simulink library "vmc"  (R2021b)
settings: Solver=VariableStepAuto  StartTime=0.0  StopTime=10.0  RelTol=1e-3
undefined symbols (not defined in the file): AVMC_ACCDeltaTqGradeGn_X_deg, AVMC_ACCDeltaTqIGain4OVRD_X_kph, AVMC_ACCDeltaTqIGain4OVRD_Y_mps2, AVMC_ACCDeltaTqIGain_X_kph, AVMC_ACCDeltaTqIGain_Y_mps2, AVMC_ACCDeltaTqPGain_X_kph, AVMC_ACCDeltaTqPGain_Y_kph, AVMC_ACCGradeofst_X_G, AVMC_ACCGradeofst_Y_pct, AVMC_ACCLoSpdTqLoLim4JP_X_kph, AVMC_ACCLoSpdTqLoLim4JP_Y_deg, AVMC_ACCLoSpdTqLowerLim_X_kph, AVMC_ACCLoSpdTqLowerLim_Y_deg, AVMC_ACCReqAccelGain_X_mps2, AVMC_ACCReqAccelGain_Y_enum, AVMC_ADSPosGFBDeltaTq_X_kph, AVMC_ADSPosGFBDeltaTq_Y_mps2, AVMC_AggressJerkPCT4AT_X_kph, AVMC_AggressJerkPCT_X_kph, AVMC_AggressLimitPCT4AT_X_kph, AVMC_AggressLimitPCT_X_kph, AVMC_DECGradeofst_X_G, AVMC_DECGradeofst_Y_pct, AVMC_DISCDeltaTqIGain_X_kph, AVMC_DISCDeltaTqIGain_Y_mps2, AVMC_DISCDeltaTqPGain_X_kph, AVMC_DISCDeltaTqPGain_Y_kph, AVMC_EPSForceSelect_X_enum, AVMC_EPSForceSelect_Y_enum, AVMC_EPSForceSelectD21_X_enum, AVMC_EPSForceSelectD21_Y_enum, AVMC_ESCRegenOut_X_kph, AVMC_ESCRegenOut_Y_Deg, AVMC_ESCRegenOutEnSpd_X_Deg, AVMC_EstPitchSlopeTs_X_kph, AVMC_GradeCompFlt_X_kph, AVMC_GyroYBandLo_X_Gps, AVMC_HoldResTq_X_kph, AVMC_ISOAccLimit_X_mps, AVMC_ISODecLimit_X_mps, AVMC_ISOJerk_X_mps, AVMC_LatESCRegenOut_X_kph, AVMC_LatESCRegenOut_Y_Deg, AVMC_LongAccDeadZone_X_kph, AVMC_LongAccFiltTsforP2_X_Gps, AVMC_MCPresBaseTq_X_bar, AVMC_MSAPedalOvrd_X_kph, AVMC_MSASpdBand_X_kph, AVMC_MSATqDownEndTq_X_kph, AVMC_MSATqDownTime_X_kph, AVMC_NegZCHoldTq_X_kph, AVMC_OPDDisSlideRate_X_Deg, AVMC_OVRD2ActSR2FCMCMD_X_mps2, AVMC_PedalTqRWhlRatio_X_Nm, AVMC_PedalTqRWhlRatio_Y_gps, AVMC_PedalTqRWhlSlipGain_X_rat, AVMC_PedalTqRWhlSlipGain_Y_kph, AVMC_PedalTqRWhSTRGGain_X_deg, AVMC_PedalTqRWhSTRGGain_Y_kph, AVMC_PosZCHoldTq_X_kph ... (+593)
libraries: hcu_lib x143, simulink x96, tqr x4, $bdroot x1, simulink_extras x1
(part 4 of 17)

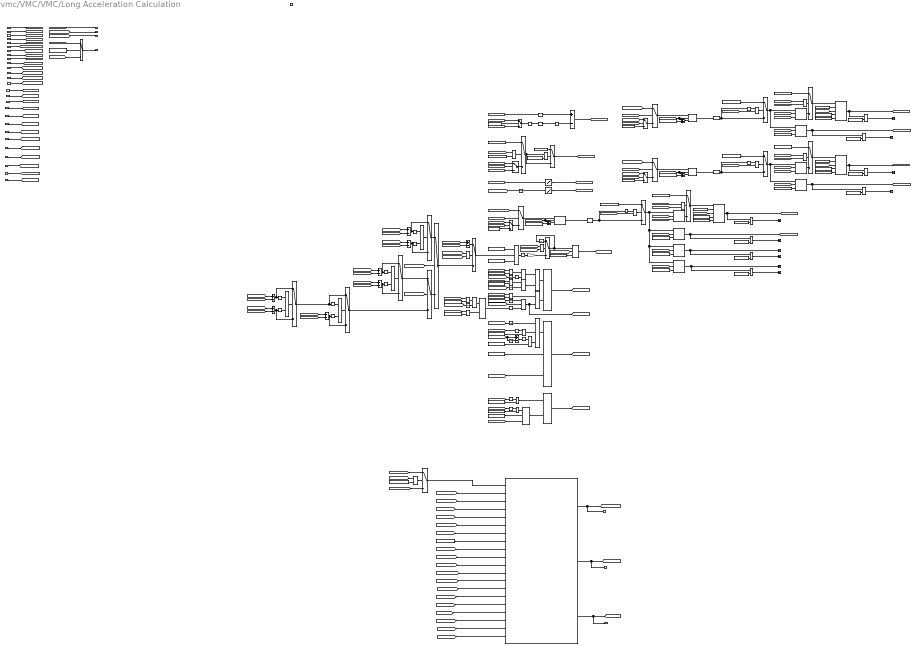
== system vmc/VMC/VMC/Long Acceleration Calculation ==
  VINP_GRADE_Deg : Inport
  VINP_LongAccel_Gps : Inport  Port=2
  VVMC_VehicleSpeed_kph : Inport  Port=3
  task_time_s : Inport  Port=4
  VVMC_EstSlopeCal_Deg : Inport  Port=5
  VVMC_LongAccelCalcuByVehSpdRaw_gps : Inport  Port=6
  VINP_DIDGetDynoMode_flg : Inport  Port=7
  VDDM_ESC5Err_flg : Inport  Port=8
  VINP_LongAccelV_flg : Inport  Port=9
  VINP_ACCRequiredAccel_mps2 : Inport  Port=10
  VVMC_LongAccelCalcuFrWhlRaw_gps : Inport  Port=11
  VVMC_LongAccelCalcuRrWhlRaw_gps : Inport  Port=12
  VVMC_FrWhlSpdInvalid_flg : Inport  Port=13
  VVMC_RrWhlSpdInvalid_flg : Inport  Port=14
  VVMC_CalibratedGyroY_Dps : Inport  Port=15
  VVMC_CalibratedAccX_G : Inport  Port=16
  VVMC_CalibratedAccY_G : Inport  Port=17
  VVMC_CalibratedAccZ_G : Inport  Port=18
  VINP_BrkPedalPos_pct : Inport  Port=19
  VTQD_GearActualPosn_enum : Inport  Port=20
  VDHP_ActAPSPosn_pct : Inport  Port=21
  VTQD_RegenMode_enum : Inport  Port=22
  VTQD_VehActSpd_kph : Inport  Port=23
  VTQD_PreLoadPreEn_flg : Inport  Port=24
  VTQR_RrTMTqReq_Nm : Inport  Port=25
  VTQR_FrTMTqReq_Nm : Inport  Port=26
  VPMM_DrivetrainSelect_enum : Inport  Port=27
  function : TriggerPort  TriggerType=function-call  VariantControl=(inherit)
  AND : Logic  Inputs=3  AllPortsSameDT=off  OutDataTypeStr=boolean
  AND1 : Logic  Operator=OR  AllPortsSameDT=off  OutDataTypeStr=boolean
  AND{2,5..8} (5 alike) : Logic  AllPortsSameDT=off  OutDataTypeStr=boolean
  AND3 : Logic  Operator=OR  AllPortsSameDT=off  OutDataTypeStr=boolean
  AND4 : Logic  Inputs=3  AllPortsSameDT=off  OutDataTypeStr=boolean
  Abs{,1..14} (15 alike) : Abs
  Add{,1..2,5..8,10..12} (10 alike) : Sum  Inputs=+-
  Add3 : Sum
  Add4 : Sum
  Add9 : Sum
  Asin1 : Trigonometry  Operator=asin
  Cast To Single{,1..4} (5 alike) : DataTypeConversion  OutDataTypeStr=single
  Constant : Constant  Value=KVMC_GradeSourceSW_flg
  Constant{1,8,17,22,24..25,33,36..37,40..41,44,47..48} (14 alike) : Constant  Value=ZERO_FLOAT
  Constant10 : Constant  Value=KVMC_LongAccelIncSRLim_gps2
  Constant11 : Constant  Value=KVMC_LongAccelDecSRLim_gps2
  Constant12 : Constant  Value=KVMC_EstSlopeFreezeSpd_kph
  Constant13 : Constant  Value=KVMC_EstSlopeUnFreezeSpd_kph
  Constant14 : Constant  Value=KVMC_EstSlopeTs_c
  Constant15 : Constant  Value=KVMC_EstSlope0SpdFreezeTime_s
  Constant16 : Constant  Value=KVMC_EstSlopeFreezeSpd_kph
  Constant18 : Constant  Value=KVMC_LongAccel0Boundary_Gps
  Constant19 : Constant  Value=KVMC_DIDGetDynoModeSW_flg
  Constant2 : Constant  Value=KVMC_AccBWFilCOFreqLo_raw32
  Constant20 : Constant  Value=KVMC_IMUGxStableThrs_Gps
  Constant21 : Constant  Value=KVMC_LongAccelSWSpd_kph
  Constant23 : Constant  Value=KVMC_GradeInvalidValue_deg
  Constant26 : Constant  Value=KVMC_EstSlopeUnFreezeSpd_kph
  Constant27 : Constant  Value=KVMC_AccBWFilterCutOffFreq_raw32
  Constant28 : Constant  Value=MINUSONE_FLOAT
  Constant29 : Constant  Value=ONE_FLOAT
  Constant3 : Constant  Value=KVMC_AccBWFilCOFreqMed_raw32
  Constant30 : Constant  Value=KVMC_EstSlopeFreezeAccel_Gps
  Constant31 : Constant  Value=KVMC_EstSlopeUnFreezeAccel_Gps
  Constant32 : Constant  Value=KVMC_EstSlopeAclUnFreezeTime_s
  Constant34 : Constant  Value=KVMC_LongAccelIncSRLim_gps2
  Constant35 : Constant  Value=KVMC_LongAccelDecSRLim_gps2
  Constant38 : Constant  Value=KVMC_AccBWFilterCutOffFreq_raw32
  Constant{5..7,9,39,46,50,52} (8 alike) : Constant  Value=KVMC_GravityValue_mps2
  Constant4 : Constant  Value=KVMC_AccBWFilCOFreqHigh_raw32
  Constant42 : Constant  Value=KVMC_LongAccelIncSRLim_gps2
  Constant43 : Constant  Value=KVMC_LongAccelDecSRLim_gps2
  Constant45 : Constant  Value=KVMC_AccBWFilterCutOffFreq_raw32
  Constant49 : Constant  Value=KVMC_AccBWFilCOFreqLo_raw32
  Constant51 : Constant  Value=KVMC_AccBWFilCOFreqLo_raw32
  Constant53 : Constant  Value=KVMC_EstSlopeGxSource_flg
  Constant54 : Constant  Value=C_TASK_10MS_S
  Constant55 : Constant  Value=KVMC_GradeTest_flg
  Degrees to Radians1 : simulink_extras/Transformations/Degrees to Radians
  DelayEnable : hcu_lib/Basic_Blocks/DelayEnable
  DelayEnable1 : hcu_lib/Basic_Blocks/DelayEnable
  Estimate Slope1 : Subsystem
  FirstOrderFilter{,1..11} (12 alike) : hcu_lib/Basic_Blocks/FirstOrderFilter
  Gain1 : Gain  Gain=RAD2DEG
  Logical Operator : Logic  Operator=OR  AllPortsSameDT=off  OutDataTypeStr=boolean
  Logical Operator1 : Logic  Operator=OR  AllPortsSameDT=off  OutDataTypeStr=boolean
  Logical Operator2 : Logic  Operator=OR  AllPortsSameDT=off  OutDataTypeStr=boolean
  MVMC_LongAccDeadZone_Y_Gps : Lookup_n-D  NumberOfTableDimensions=1  BreakpointsForDimension1=AVMC_LongAccDeadZone_X_kph  Table=MVMC_LongAccDeadZone_Y_Gps  InternalRulePriority=Speed  RndMeth=Simplest  InputSameDT=on
  MVMC_LongAccFiltTsforP2_Y_c : Lookup_n-D  NumberOfTableDimensions=1  BreakpointsForDimension1=AVMC_LongAccFiltTsforP2_X_Gps  Table=MVMC_LongAccFiltTsforP2_Y_c  InternalRulePriority=Speed  RndMeth=Simplest  InputSameDT=on
  NOT1 : Logic  Operator=NOT  AllPortsSameDT=off  OutDataTypeStr=boolean
  NOT2 : Logic  Operator=NOT  AllPortsSameDT=off  OutDataTypeStr=boolean
  OR : Logic  Operator=OR  AllPortsSameDT=off  OutDataTypeStr=boolean
  OR21 : Logic  AllPortsSameDT=off  OutDataTypeStr=boolean
  Product{1..7,15} (8 alike) : Product
  RateLimit1 : tqr/TQR/Determine Torque Request/TorqueArbitrament/TorqueSmooth/RateLimit
  RateLimit2 : tqr/TQR/Determine Torque Request/TorqueArbitrament/TorqueSmooth/RateLimit
  RateLimit3 : tqr/TQR/Determine Torque Request/TorqueArbitrament/TorqueSmooth/RateLimit
  Relational Operator : RelationalOperator  Operator=>  OutDataTypeStr=boolean  RndMeth=Simplest
  Relational Operator{1,4,7,10} (4 alike) : RelationalOperator  Operator=<  OutDataTypeStr=boolean  RndMeth=Simplest
  Relational Operator{2,5..6,11..12,124..127} (9 alike) : RelationalOperator  Operator=<=  OutDataTypeStr=boolean  RndMeth=Simplest
  Relational Operator3 : RelationalOperator  OutDataTypeStr=boolean  RndMeth=Simplest
  Relational Operator8 : RelationalOperator  OutDataTypeStr=boolean  RndMeth=Simplest
  Relational Operator9 : RelationalOperator  OutDataTypeStr=boolean  RndMeth=Simplest
  SR_Latch : hcu_lib/Basic_Blocks/SR_Latch
  SR_Latch1 : hcu_lib/Basic_Blocks/SR_Latch
  SR_Latch2 : hcu_lib/Basic_Blocks/SR_Latch
  Saturation Dynamic3 : simulink/Discontinuities/Saturation Dynamic  OutMin=[]  OutMax=[]  OutDataTypeStr=Inherit: Same as second input  OutDataType=fixdt(1, 16)  OutScaling=2^-10  DoSatur=off
  Sin1 : Trigonometry
  Switch{,1..4,6..8,10,12..14,16..17,82..83,85..89} (21 alike) : Switch  Criteria=u2 > Threshold
  Switch{5,9,11,15} (4 alike) : Switch  Criteria=u2 > Threshold  Threshold=KVMC_LongAccelSWSpd_kph
  Switch18 : Switch  Criteria=u2 ~= 0
      settings: AttributesFormatString=%<Criteria>
  Terminator{1..7,9..11} (10 alike) : Terminator
  Unit Delay{,1..7} (8 alike) : UnitDelay  SampleTime=-1  HasFrameUpgradeWarning=on
  VVMC_LongAcc_Gps : Outport
  VVMC_EstSlope_Deg : Outport  Port=2
  VVMC_LongAccFrWhl_Gps : Outport  Port=3
  VVMC_LongAccRrWhl_Gps : Outport  Port=4
  VVMC_EstSlopeCalBase_Deg : Outport  Port=5
  VVMC_IMUEstSlope_Deg1 : Outport  Port=6
  VVMC_FinalSlop_deg : Outport  Port=7
  wires:
  Switch/1 -> Degrees to Radians1/1
  AND5/1 -> Switch16/2
  VDDM_ESC5Err_flg/1 -> [VDDM_ESC5Err_flg]
  [VVMC_LongAccDeadZone_Gps] -> Relational Operator2/2
  Constant/1 -> Switch/2
  VVMC_VehicleSpeed_kph/1 -> [VVMC_VehicleSpeed_kph]
  Cast To Single/1 -> Sin1/1  "VVMC_GRADE_rad"
  [VVMC_VehicleSpeed_kph] -> MVMC_LongAccDeadZone_Y_Gps/1
  Abs/1 -> Relational Operator2/1
  VVMC_EstSlopeCal_Deg/1 -> [VVMC_EstSlopeCal_Deg]
  [VDDM_ESC5Err_flg] -> Logical Operator/1
  Relational Operator2/1 -> Switch1/2
  task_time_s/1 -> [task_time_s]
  Constant17/1 -> Switch14/3
  VINP_GRADE_Deg/1 -> [VINP_GRADE_Deg]
  [VINP_LongAccel_Gps] -> Cast To Single1/1
  [VVMC_LongAccFiltTsforP2_c] -> FirstOrderFilter/3
  Switch17/1 -> [VVMC_InitEstSlope_Deg]  "VVMC_InitEstSlope_Deg"
  RateLimit1/1 -> [VVMC_LongAcc_Gps], Product2/1  "VVMC_LongAcc_Gps"
  Degrees to Radians1/1 -> Cast To Single/1
  MVMC_LongAccFiltTsforP2_Y_c/1 -> [VVMC_LongAccFiltTsforP2_c]  "VVMC_LongAccFiltTsforP2_c"
  [VINP_DIDGetDynoMode_flg] -> AND5/1
  Switch1/1 -> FirstOrderFilter/1, FirstOrderFilter1/1, FirstOrderFilter3/1, FirstOrderFilter2/1
  [VVMC_VehicleSpeed_kph] -> Switch11/2
  VVMC_LongAccelCalcuByVehSpdRaw_gps/1 -> [VVMC_LongAccelCalcuByVehSpdRaw_gps]
  [VVMC_LongAcc_Gps] -> VVMC_LongAcc_Gps/1
  [task_time_s] -> FirstOrderFilter8/2, Add9/1
  [task_time_s] -> FirstOrderFilter/2
  Add9/1 -> FirstOrderFilter8/3
  [VINP_GRADE_Deg] -> Switch/1
  [VVMC_LongAccCal1_Gps] -> Switch14/1
  [VVMC_VehicleSpeed_kph] -> Switch15/2
  Switch14/1 -> Switch11/3
  [VVMC_VehicleSpeed_kph] -> Switch14/2
  FirstOrderFilter/1 -> Switch2/3
  VINP_DIDGetDynoMode_flg/1 -> [VINP_DIDGetDynoMode_flg]
  Constant23/1 -> Relational Operator/2
  Cast To Single1/1 -> Add2/1
  VINP_LongAccel_Gps/1 -> [VINP_LongAccel_Gps]
  [VVMC_EstSlopeCal_Deg] -> Switch15/1
  Relational Operator/1 -> Switch17/2
  MVMC_LongAccDeadZone_Y_Gps/1 -> [VVMC_LongAccDeadZone_Gps]  "VVMC_LongAccDeadZone_Gps"
  [VINP_GRADE_Deg] -> Switch15/3
  Switch16/1 -> Switch17/3, Relational Operator/1
  Switch11/1 -> FirstOrderFilter8/1
  Constant27/1 -> Add9/2
  Constant22/1 -> Switch16/1
  Constant25/1 -> Switch2/1
  Add2/1 -> [VVMC_LongAccCal1_Gps]  "VVMC_LongAccCal1_Gps"
  Switch15/1 -> Switch16/3
  Constant24/1 -> Switch17/1
  [VINP_LongAccelV_flg] -> Logical Operator/2
  Constant1/1 -> Switch1/1
  Cast To Single2/1 -> Abs/1, Switch1/3
  Sin1/1 -> Add2/2  "VVMC_SINEGRADE_Gps"
  VINP_LongAccelV_flg/1 -> [VINP_LongAccelV_flg]
  Logical Operator/1 -> Switch2/2
  [VVMC_InitEstSlope_Deg] -> Switch/3
  FirstOrderFilter8/1 -> Cast To Single2/1  "VVMC_LongAccelCalcuByVehSpd_gps"
  [VVMC_LongAccelCalcuByVehSpdRaw_gps] -> Switch11/1
  Constant19/1 -> AND5/2
  [task_time_s] -> FirstOrderFilter1/2
  Constant2/1 -> FirstOrderFilter1/3
  Constant3/1 -> FirstOrderFilter2/3
  [task_time_s] -> FirstOrderFilter2/2
  FirstOrderFilter1/1 -> [VVMC_LongAccLowFilt_Gps], Product1/1  "VVMC_LongAccLowFilt_Gps"
  FirstOrderFilter2/1 -> Terminator2/1, Product3/1  "VVMC_LongAccMedFilt_Gps"
  FirstOrderFilter3/1 -> Terminator4/1, Product4/1  "VVMC_LongAccHighFilt_Gps"
  [task_time_s] -> FirstOrderFilter3/2
  Constant4/1 -> FirstOrderFilter3/3
  Constant9/1 -> Product1/2
  Product1/1 -> Terminator1/1  "VVMC_LongAccLowFilt_mps2"
  Constant5/1 -> Product2/2
  Product2/1 -> Terminator6/1  "VVMC_LongAcc_mps2"
  Product3/1 -> Terminator3/1  "VVMC_LongAccMedFilt_mps2"
  Constant6/1 -> Product3/2
  Constant7/1 -> Product4/2
  Product4/1 -> Terminator5/1  "VVMC_LongAccHighFilt_mps2"
  VINP_ACCRequiredAccel_mps2/1 -> [VINP_ACCRequiredAccel_mps2]
  [VINP_ACCRequiredAccel_mps2] -> Unit Delay/1
  Unit Delay/1 -> MVMC_LongAccFiltTsforP2_Y_c/1
  Constant11/1 -> RateLimit1/5
  Constant10/1 -> RateLimit1/4
  [task_time_s] -> RateLimit1/3
  Constant8/1 -> RateLimit1/2
  Switch2/1 -> RateLimit1/1
  [VVMC_EstSlopeFreezeEn_flg] -> Unit Delay2/1
  Saturation Dynamic3/1 -> Asin1/1
  Constant28/1 -> Saturation Dynamic3/3
  [VVMC_VehicleSpeed_kph] -> Relational Operator8/1
  Abs1/1 -> Relational Operator5/1
  Constant29/1 -> Saturation Dynamic3/1
  SR_Latch1/1 -> NOT2/1  "VVMC_EstSlope0SpdUnFrzOnce_flg"
  AND7/1 -> SR_Latch1/1
  DelayEnable/1 -> [VVMC_EstSlopeLowSpdGxStable_flg]  "VVMC_EstSlopeLowSpdGxStable_flg"
  Relational Operator5/1 -> AND4/2
  AND6/1 -> AND3/2
  Constant26/1 -> Relational Operator8/2
  NOT2/1 -> AND/3
  Relational Operator3/1 -> AND1/1
  Unit Delay7/1 -> AND7/2
  [VVMC_EstSlopeLowSpdUnFreeze_flg] -> Unit Delay7/1
  [VINP_LongAccel_Gps] -> Add/1, Unit Delay6/1
  [VVMC_VehicleSpeed_kph] -> Relational Operator7/1
  Unit Delay6/1 -> Add/2
  [VINP_LongAccel_Gps] -> Add1/1
  Constant18/1 -> Relational Operator5/2
  Constant16/1 -> Relational Operator4/2
  Unit Delay1/1 -> Switch3/1
  Switch82/1 -> Saturation Dynamic3/2
  Abs2/1 -> Relational Operator6/1
  Constant21/1 -> Relational Operator7/2
  Constant20/1 -> Relational Operator6/2
  Add/1 -> Abs2/1
  Unit Delay5/1 -> AND4/1
  Unit Delay2/1 -> AND/1
  Relational Operator8/1 -> SR_Latch1/2
  Unit Delay3/1 -> NOT1/1
  SR_Latch/1 -> [VVMC_EstSlopeFreezeEn_flg]  "VVMC_EstSlopeFreezeEn_flg"
  AND/1 -> AND1/2, [VVMC_EstSlopeLowSpdUnFreeze_flg]  "VVMC_EstSlopeLowSpdUnFreeze_flg"
  Relational Operator7/1 -> AND7/1
  AND2/1 -> AND3/1
  [VVMC_EstSlopeLowSpdUnFreeze_flg] -> Unit Delay3/1
  [VVMC_EstSlopeFreezeEn_flg] -> Unit Delay5/1
  Relational Operator6/1 -> AND4/3
  [VVMC_VehicleSpeed_kph] -> Relational Operator1/1
  [VVMC_EstSlopeFreezeEn_flg] -> OR/1
  NOT1/1 -> AND2/2
  AND3/1 -> SR_Latch/1
  Constant15/1 -> DelayEnable/2
  Switch3/1 -> Unit Delay1/1, FirstOrderFilter5/1
  Gain1/1 -> Switch3/3
  [VVMC_LongAccLowFilt_Gps] -> Abs1/1
  [VVMC_VehicleSpeed_kph] -> Relational Operator4/1
  Constant14/1 -> FirstOrderFilter5/3
  Asin1/1 -> Gain1/1
  Relational Operator4/1 -> AND6/1
  Constant13/1 -> Relational Operator3/2
  FirstOrderFilter5/1 -> [VVMC_HoldEstSlope_deg]  "VVMC_HoldEstSlope_deg"
  [VVMC_EstSlopeLowSpdGxStable_flg] -> AND/2
  [task_time_s] -> DelayEnable/3
  [VVMC_EstSlopeLowSpdUnFreeze_flg] -> Unit Delay4/1
  Unit Delay4/1 -> AND6/2
  AND1/1 -> SR_Latch/2
  [task_time_s] -> FirstOrderFilter5/2
  Constant12/1 -> Relational Operator1/2
  [VVMC_VehicleSpeed_kph] -> Relational Operator3/1
  Relational Operator1/1 -> AND2/1
  AND4/1 -> DelayEnable/1
  [VVMC_LongAccLowFilt_Gps] -> Abs3/1
  Abs3/1 -> Relational Operator9/1
  Constant30/1 -> Relational Operator9/2
  Relational Operator9/1 -> SR_Latch2/1
  DelayEnable1/1 -> SR_Latch2/2
  [task_time_s] -> DelayEnable1/3
  Relational Operator10/1 -> DelayEnable1/1
  [VVMC_LongAccLowFilt_Gps] -> Abs4/1
  Constant31/1 -> Relational Operator10/2
  Constant32/1 -> DelayEnable1/2
  SR_Latch2/1 -> [VVMC_EstSlopeAclFreezeEn_flg]  "VVMC_EstSlopeAclFreezeEn_flg"
  Abs4/1 -> Relational Operator10/1
  OR/1 -> Switch3/2
  [VVMC_EstSlopeAclFreezeEn_flg] -> OR/2
  VVMC_LongAccelCalcuFrWhlRaw_gps/1 -> [VVMC_LongAccelCalcuFrWhlRaw_gps]
  VVMC_LongAccelCalcuRrWhlRaw_gps/1 -> [VVMC_LongAccelCalcuRrWhlRaw_gps]
  [task_time_s] -> RateLimit2/3
  Switch7/1 -> RateLimit2/1
  Product5/1 -> Terminator7/1  "VVMC_LongAccFrWhl_mps2"
  Constant35/1 -> RateLimit2/5
  [task_time_s] -> FirstOrderFilter6/2, Add3/1
  [VVMC_LongAccDeadZone_Gps] -> Relational Operator11/2
  Constant33/1 -> Switch4/1
  Cast To Single3/1 -> Switch4/3, Abs5/1
  [VVMC_LongAccelCalcuFrWhlRaw_gps] -> Switch5/1
  FirstOrderFilter6/1 -> Cast To Single3/1  "VVMC_LongAccelCalcuFrWhl_gps"
  Switch6/1 -> Switch5/3
  Constant37/1 -> Switch7/1
  Constant38/1 -> Add3/2
  [VINP_LongAccelV_flg] -> Logical Operator1/2
  [VVMC_LongAccFiltTsforP2_c] -> FirstOrderFilter4/3
  RateLimit2/1 -> [VVMC_LongAccFrWhl_Gps], Product5/1  "VVMC_LongAccFrWhl_Gps"
  Abs5/1 -> Relational Operator11/1
  [VDDM_ESC5Err_flg] -> Logical Operator1/1
  Constant39/1 -> Product5/2
  Constant36/1 -> Switch6/3
  Constant34/1 -> RateLimit2/4
  FirstOrderFilter4/1 -> Switch7/3
  Constant40/1 -> RateLimit2/2
  [VVMC_LongAccCal1_Gps] -> Switch6/1
  Relational Operator11/1 -> Switch4/2
  Switch5/1 -> FirstOrderFilter6/1
  [VVMC_VehicleSpeed_kph] -> Switch6/2
  Switch4/1 -> FirstOrderFilter11/1, FirstOrderFilter4/1
  [VVMC_VehicleSpeed_kph] -> Switch5/2
  Logical Operator1/1 -> Switch7/2
  Add3/1 -> FirstOrderFilter6/3
  [task_time_s] -> FirstOrderFilter4/2
  [task_time_s] -> FirstOrderFilter7/2
  Add4/1 -> FirstOrderFilter9/3
  Logical Operator2/1 -> Switch12/2
  [VVMC_VehicleSpeed_kph] -> Switch9/2
  Switch8/1 -> FirstOrderFilter10/1, FirstOrderFilter7/1
  [VVMC_VehicleSpeed_kph] -> Switch10/2
  Switch9/1 -> FirstOrderFilter9/1
  Relational Operator12/1 -> Switch8/2
  [VVMC_LongAccCal1_Gps] -> Switch10/1
  Constant47/1 -> RateLimit3/2
  FirstOrderFilter7/1 -> Switch12/3
  Constant42/1 -> RateLimit3/4
  Constant44/1 -> Switch10/3
  Constant46/1 -> Product6/2
  [VDDM_ESC5Err_flg] -> Logical Operator2/1
  Abs6/1 -> Relational Operator12/1
  RateLimit3/1 -> Product6/1, [VVMC_LongAccRrWhl_Gps]  "VVMC_LongAccRrWhl_Gps"
  [VVMC_LongAccFiltTsforP2_c] -> FirstOrderFilter7/3
  [VINP_LongAccelV_flg] -> Logical Operator2/2
  Constant45/1 -> Add4/2
  Switch10/1 -> Switch9/3
  FirstOrderFilter9/1 -> Cast To Single4/1  "VVMC_LongAccelCalcuRrWhl_gps"
  [VVMC_LongAccelCalcuRrWhlRaw_gps] -> Switch9/1
  Cast To Single4/1 -> Abs6/1, Switch8/3
  Constant41/1 -> Switch8/1
  [VVMC_LongAccDeadZone_Gps] -> Relational Operator12/2
  [task_time_s] -> Add4/1, FirstOrderFilter9/2
  Constant43/1 -> RateLimit3/5
  Product6/1 -> Terminator9/1  "VVMC_LongAccRrWhl_mps2"
  Switch12/1 -> RateLimit3/1
  [task_time_s] -> RateLimit3/3
  [VVMC_LongAccFrWhl_Gps] -> VVMC_LongAccFrWhl_Gps/1
  [VVMC_LongAccRrWhl_Gps] -> VVMC_LongAccRrWhl_Gps/1
  Constant48/1 -> Switch12/1
  Abs10/1 -> Relational Operator125/2
  Abs11/1 -> Relational Operator126/1
  Add6/1 -> Switch86/3, Abs8/1
  Switch89/1 -> Switch85/3
  Relational Operator127/1 -> Switch89/2
  [VVMC_FrWhlSpdInvalid_flg] -> Switch83/2
  Abs14/1 -> Relational Operator127/2
  Add10/1 -> Switch89/3, Abs14/1
  Abs13/1 -> Relational Operator127/1
  Add11/1 -> Abs11/1, Switch88/1
  [VVMC_FrWhlSpdInvalid_flg] -> OR21/1
  Relational Operator126/1 -> Switch88/2
  Switch88/1 -> Switch89/1, Abs13/1
  Relational Operator125/1 -> Switch87/2
  Add8/1 -> Abs10/1, Switch87/3
  [VVMC_RrWhlSpdInvalid_flg] -> OR21/2
  Abs9/1 -> Relational Operator125/1
  Add12/1 -> Abs12/1, Switch88/3
  Switch86/1 -> Switch83/1
  Switch85/1 -> Switch83/3
  Relational Operator124/1 -> Switch86/2
  Abs8/1 -> Relational Operator124/2
  Add5/1 -> Switch86/1, Abs7/1
  Abs7/1 -> Relational Operator124/1
  [VVMC_LongAccLowFilt_Gps] -> Add1/2
  Switch83/1 -> Switch82/3
  Abs12/1 -> Relational Operator126/2
  [VVMC_RrWhlSpdInvalid_flg] -> Switch85/2
  Switch87/1 -> Switch85/1
  Add7/1 -> Abs9/1, Switch87/1
  OR21/1 -> Switch82/2
  FirstOrderFilter10/1 -> [VVMC_LongAccRrWhlLowFilt_Gps], Product7/1  "VVMC_LongAccRrWhlLowFilt_Gps"
  Constant50/1 -> Product7/2
  Product7/1 -> Terminator10/1  "VVMC_LongAccRrWhlLowFilt_mps2"
  Constant49/1 -> FirstOrderFilter10/3
  [task_time_s] -> FirstOrderFilter10/2
  [task_time_s] -> FirstOrderFilter11/2
  Constant51/1 -> FirstOrderFilter11/3
  Product15/1 -> Terminator11/1  "VVMC_LongAccFrWhlLowFilt_mps2"
  Constant52/1 -> Product15/2
  FirstOrderFilter11/1 -> Product15/1, [VVMC_LongAccFrWhlLowFilt_Gps]  "VVMC_LongAccFrWhlLowFilt_Gps"
  Add1/1 -> Switch82/1
  [VINP_LongAccel_Gps] -> Add5/1
  [VVMC_LongAccLowFilt_Gps] -> Add5/2
  [VINP_LongAccel_Gps] -> Add6/1
  [VVMC_LongAccRrWhlLowFilt_Gps] -> Add6/2
  [VVMC_LongAccLowFilt_Gps] -> Add7/2
  [VINP_LongAccel_Gps] -> Add7/1
  [VVMC_LongAccFrWhlLowFilt_Gps] -> Add8/2
  [VINP_LongAccel_Gps] -> Add8/1
  [VINP_LongAccel_Gps] -> Add10/1
  [VVMC_LongAccFrWhlLowFilt_Gps] -> Add10/2
  [VVMC_LongAccRrWhlLowFilt_Gps] -> Add12/2
  [VINP_LongAccel_Gps] -> Add12/1
  [VVMC_LongAccLowFilt_Gps] -> Add11/2
  [VINP_LongAccel_Gps] -> Add11/1
  VVMC_FrWhlSpdInvalid_flg/1 -> [VVMC_FrWhlSpdInvalid_flg]
  VVMC_RrWhlSpdInvalid_flg/1 -> [VVMC_RrWhlSpdInvalid_flg]
  Constant53/1 -> AND8/2
  [VTQD_VehActSpd_kph] -> Estimate Slope1/13(VTQD_VehActSpd_kph)
  AND8/1 -> Switch13/2
  [VINP_GRADE_deg] -> Estimate Slope1/3(VINP_GRADE_deg)
  Estimate Slope1/2(VVMC_IMUEstSlope_Deg1) -> VVMC_IMUEstSlope_Deg1/1, [VVMC_IMUEstSlope_Deg1]
  [VINP_BrkPedalPos_pct] -> Estimate Slope1/12(VINP_BrkPedalPos_pct)
  [VDHP_ActAPSPosn_pct] -> Estimate Slope1/9(VDHP_ActAPSPosn_pct)
  [VVMC_CalibratedGyroY_Dps] -> Estimate Slope1/4(VVMC_CalibratedGyroY_Dps)
  [VVMC_CalibratedAccZ_G] -> Estimate Slope1/7(VVMC_CalibratedAccZ_G)
  Switch13/1 -> Estimate Slope1/1(VINP_LongAccel_Gps)
  [VTQD_RegenMode_enum] -> Estimate Slope1/14(VTQD_RegenMode_enum)
  Constant54/1 -> Estimate Slope1/8(C_TASK_10MS_S)
  [VVMC_VehicleSpeed_kph] -> Estimate Slope1/2(VINP_VehSpeed_kph)
  Estimate Slope1/1(VVMC_EstSlopeCalBase_Deg) -> VVMC_EstSlopeCalBase_Deg/1, [VVMC_EstSlopeCalBase_Deg]
  [VVMC_CalibratedAccX_G] -> Estimate Slope1/5(VVMC_CalibratedAccX_G)
  [VVMC_CalibratedAccY_G] -> Estimate Slope1/6(VVMC_CalibratedAccY_G)
  [VINP_LongAccel_Gps] -> Switch13/3
  Estimate Slope1/3(VVMC_FinalSlop_deg) -> VVMC_FinalSlop_deg/1, [VVMC_FinalSlop_deg]
  [VVMC_CalibratedAccX_G] -> Switch13/1
  [VTQD_PreLoadPreEn_flg] -> Estimate Slope1/11(VTQD_PreLoadPreEn_flg)
  [VINP_DIDGetDynoMode_flg] -> Estimate Slope1/15(VINP_DIDGetDynoMode_flg)
  [VTQD_GearActualPosn_enum] -> Estimate Slope1/10(VTQD_GearActualPosn_enum)
  [VVMC_IMUEnaCmd_flg] -> AND8/1
  VVMC_CalibratedGyroY_Dps/1 -> [VVMC_CalibratedGyroY_Dps]
  VVMC_CalibratedAccX_G/1 -> [VVMC_CalibratedAccX_G]
  VVMC_CalibratedAccY_G/1 -> [VVMC_CalibratedAccY_G]
  VVMC_CalibratedAccZ_G/1 -> [VVMC_CalibratedAccZ_G]
  VINP_BrkPedalPos_pct/1 -> [VINP_BrkPedalPos_pct]
  VTQD_GearActualPosn_enum/1 -> [VTQD_GearActualPosn_enum]
  VDHP_ActAPSPosn_pct/1 -> [VDHP_ActAPSPosn_pct]
  VTQD_RegenMode_enum/1 -> [VTQD_RegenMode_enum]
  VTQD_VehActSpd_kph/1 -> [VTQD_VehActSpd_kph]
  VTQD_PreLoadPreEn_flg/1 -> [VTQD_PreLoadPreEn_flg]
  [VVMC_HoldEstSlope_deg] -> Estimate Slope1/16(VVMC_HoldEstSlope_deg)
  [VVMC_InitEstSlope_Deg] -> Estimate Slope1/17(VVMC_InitEstSlope_Deg)
  VTQR_RrTMTqReq_Nm/1 -> [VTQR_RrTMTqReq_Nm]
  VTQR_FrTMTqReq_Nm/1 -> [VTQR_FrTMTqReq_Nm]
  VPMM_DrivetrainSelect_enum/1 -> [VPMM_DrivetrainSelect_enum]
  [VTQR_RrTMTqReq_Nm] -> Estimate Slope1/18(VTQR_RrTMTqReq_Nm)
  [VTQR_FrTMTqReq_Nm] -> Estimate Slope1/19(VTQR_FrTMTqReq_Nm)
  [VPMM_DrivetrainSelect_enum] -> Estimate Slope1/20(VPMM_DrivetrainSelect_enum)
  [VVMC_FinalSlop_deg] -> Switch18/3
  Constant55/1 -> Switch18/2
  [VVMC_InitEstSlope_Deg] -> Switch18/1
  Switch18/1 -> VVMC_EstSlope_Deg/1  "VVMC_EstSlope_Deg"

== system vmc/VMC/VMC/MSA function ==
  VTQD_ExternalTqAllow_flg : Inport
  VTQD_DriverWhlTqDem_Nm : Inport  Port=2
  <VTQD_SpdCtrlMode_enum> : Inport  Port=3
  VTQD_SWC2CANCELSta_flg : Inport  Port=4
  VVMC_VehicleSpeed_kph : Inport  Port=5
  VVMC_LongAcc_Gps : Inport  Port=6
  VVMC_FeatSetSpdForCalcu_kph : Inport  Port=7
  VVMC_FeatArbitrFinal_enum : Inport  Port=8
  VTQD_SWC2ResUpSta_flg : Inport  Port=9
  VTQD_SWC2SetdownSta_flg : Inport  Port=10
  VVMC_MeterIndSpeedForCalcu_kph : Inport  Port=11
  VTQD_LowIdleAccPedal_flg : Inport  Port=12
  VDHP_ActAPSPosn_pct : Inport  Port=13
  task_time_s : Inport  Port=14
  VVMC_ActACCRequiredAccel_mps2 : Inport  Port=15
  VTQR_FrTMTqReq_Nm : Inport  Port=16
  VTQR_RrTMTqReq_Nm : Inport  Port=17
  VVMC_TotalAvailBrkRgnTq_Nm : Inport  Port=18
  VINP_HoodSW_flg : Inport  Port=19
  VTQD_GearActualPosn_enum : Inport  Port=20
  VINP_Distanceunit_flg : Inport  Port=21
  VINP_SmartEcoModeSW_flg : Inport  Port=22
  VVMC_APSActive_flg : Inport  Port=23
  VVMC_VMCMSACtrlAvail_flg : Inport  Port=24
  VINP_SWCType_enum : Inport  Port=25
  VTQD_SWC1CANCELSta_flg : Inport  Port=26
  VTQD_SWC1ResUpSta_flg : Inport  Port=27
  VTQD_SWC1SetdownSta_flg : Inport  Port=28
  VVMC_FeatSetSpdFinal_raw32 : Inport  Port=29
  VVMC_MeterIndSpeed_raw32 : Inport  Port=30
  VINP_RDCActive_enum : Inport  Port=31
  " 2" : Constant  Value=ENUM_SWCTYPE_SWC2
  Add : Sum  Inputs=+-
  Anti-Speed Limitation : Subsystem
  Constant : Constant  Value=TRUE
  Constant1 : Constant  Value=KVMC_CCMSASpdWar_kph
  Constant3 : Constant  Value=ENUM_ADASMSASTA_OFF
  Constant6 : Constant  Value=ENUM_EXTRAMSACTRLSTA_ANTISPEEDLIMIT
  Constant7 : Constant  Value=ENUM_EXTRAMSACTRLSTA_OFF
  Data Type Conversion : DataTypeConversion  OutDataTypeStr=single
  MSAActivationHandshake : Subsystem
  MSADemandTorqueCalculation : Subsystem
  MSATorqueSourceDetermination : Subsystem
  Relational Operator : RelationalOperator  OutDataTypeStr=boolean  RndMeth=Simplest
  Relational Operator3 : RelationalOperator  Operator===  OutDataTypeStr=boolean  RndMeth=Simplest
  Switch{,1..6} (7 alike) : Switch  Criteria=u2 > Threshold
  Unit Delay : UnitDelay  SampleTime=-1  HasFrameUpgradeWarning=on
  VVMC_MSACtrlSta_enum : Outport
  VVMC_MSAWhlTqReq_Nm : Outport  Port=2
  VVMC_MSASpdWar_flg : Outport  Port=3
  VVMC_MSAActive_flg : Outport  Port=4
  VVMC_MSAWhlTqActive_flg : Outport  Port=5
  VVMC_ExtraMSACtrlSta_enum : Outport  Port=6
  VVMC_AntiLimitSpd_kph : Outport  Port=7
  VVMC_AntiSpdLimSpdEn_flg : Outport  Port=8
  wires:
  [VTQD_SWC1ResUpSta_flg] -> Switch6/3
  [VTQD_SWC2ResUpSta_flg] -> Switch6/1
  Relational Operator3/1 -> Switch6/2
  [VINP_SWCType_enum] -> Relational Operator3/1
  " 2"/1 -> Relational Operator3/2
  VVMC_FeatSetSpdFinal_raw32/1 -> [VVMC_FeatSetSpdFinal_raw32]
  [VTQD_SWC1SetdownSta_flg] -> MSAActivationHandshake/16(VTQD_SWC1SetdownSta_flg)
  [VTQD_SWC1ResUpSta_flg] -> MSAActivationHandshake/15(VTQD_SWC1ResUpSta_flg)
  [VTQD_SWC1CANCELSta_flg] -> MSAActivationHandshake/14(VTQD_SWC1CANCELSta_flg)
  VTQD_SWC1SetdownSta_flg/1 -> [VTQD_SWC1SetdownSta_flg]
  VTQD_SWC1ResUpSta_flg/1 -> [VTQD_SWC1ResUpSta_flg]
  VTQD_SWC1CANCELSta_flg/1 -> [VTQD_SWC1CANCELSta_flg]
  [VINP_SWCType_enum] -> MSAActivationHandshake/13(VINP_SWCType_enum)
  VINP_SWCType_enum/1 -> [VINP_SWCType_enum]
  [VVMC_VMCMSACtrlAvail_flg] -> MSAActivationHandshake/12(VVMC_VMCMSACtrlAvail_flg)
  VVMC_VMCMSACtrlAvail_flg/1 -> [VVMC_VMCMSACtrlAvail_flg]
  [VTQD_GearActualPosn_enum] -> MSAActivationHandshake/11(VTQD_GearActualPosn_enum)
  [VVMC_AntiSpdLimSpdEn_flg] -> VVMC_AntiSpdLimSpdEn_flg/1
  [VVMC_AntiLimitSpd_kph] -> VVMC_AntiLimitSpd_kph/1
  [VVMC_IntMSACtrlSta_enum] -> Anti-Speed Limitation/5(VVMC_IntMSACtrlSta_enum)
  [VVMC_APSActive_flg] -> Anti-Speed Limitation/4(VVMC_APSActive_flg)
  [VINP_SmartEcoModeSW_flg] -> Anti-Speed Limitation/3(VINP_SmartEcoModeSW_flg)
  Anti-Speed Limitation/4(VVMC_AntiSpdLimStaEn_flg) -> [VVMC_AntiSpdLimStaEn_flg]
  Anti-Speed Limitation/3(VVMC_AntiSpdLimSpdEn_flg) -> [VVMC_AntiSpdLimSpdEn_flg]
  Anti-Speed Limitation/2(VVMC_AntiLimitSpd_kph) -> [VVMC_AntiLimitSpd_kph]
  Anti-Speed Limitation/1(VVMC_AntiSpdLimEn_flg) -> [VVMC_AntiSpdLimEn_flg]
  VINP_SmartEcoModeSW_flg/1 -> [VINP_SmartEcoModeSW_flg]
  VVMC_APSActive_flg/1 -> [VVMC_APSActive_flg]
  [VVMC_ExtraMSACtrlSta_enum] -> VVMC_ExtraMSACtrlSta_enum/1
  Switch5/1 -> [VVMC_ExtraMSACtrlSta_enum]  "VVMC_ExtraMSACtrlSta_enum"
  Constant7/1 -> Switch5/3
  Constant6/1 -> Switch5/1
  [VVMC_AntiSpdLimEn_flg] -> Switch5/2
  VINP_Distanceunit_flg/1 -> [VINP_Distanceunit_flg]
  [VINP_Distanceunit_flg] -> MSAActivationHandshake/10(VINP_Distanceunit_flg)
  [VVMC_AntiSpdLimSpdEn_flg] -> MSATorqueSourceDetermination/11(VVMC_AntiSpdLimSpdEn_flg)
  [VVMC_FeatSetSpdForCalcu_kph] -> Switch4/3
  [VVMC_AntiSpdLimSpdEn_flg] -> Switch4/2
  [VVMC_AntiLimitSpd_kph] -> Switch4/1
  [VVMC_AntiLimitSpd_kph] -> Switch3/1
  Switch3/1 -> MSADemandTorqueCalculation/1(VVMC_FeatSetSpdForCalcu_kph)
  [VVMC_AntiSpdLimSpdEn_flg] -> Switch3/2
  MSAActivationHandshake/1(VVMC_IntMSACtrlSta_enum) -> Switch2/3, [VVMC_IntMSACtrlSta_enum]
  [VVMC_AntiSpdLimStaEn_flg] -> Switch2/2
  Constant3/1 -> Switch2/1
  Constant1/1 -> Relational Operator/2
  Add/1 -> Relational Operator/1
  [VVMC_AntiLimitSpd_kph] -> Add/2
  [VVMC_MeterIndSpeedForCalcu_kph] -> Add/1
  MSAActivationHandshake/2(VVMC_IntMSASpdWar_flg) -> Switch1/3
  [VVMC_AntiSpdLimSpdEn_flg] -> Switch1/2
  Relational Operator/1 -> Switch1/1
  Constant/1 -> Switch/1
  MSAActivationHandshake/3(VVMC_IntMSAActive_flg) -> Switch/3
  [VVMC_AntiSpdLimSpdEn_flg] -> Switch/2
  VTQD_GearActualPosn_enum/1 -> [VTQD_GearActualPosn_enum]
  [VINP_HoodSW_flg] -> Anti-Speed Limitation/1(VINP_HoodSW_flg)
  [VTQD_GearActualPosn_enum] -> Anti-Speed Limitation/2(VTQD_GearActualPosn_enum)
  VINP_HoodSW_flg/1 -> [VINP_HoodSW_flg]
  [VVMC_TotalAvailBrkRgnTq_Nm] -> MSADemandTorqueCalculation/12(VVMC_TotalAvailBrkRgnTq_Nm)
  VVMC_TotalAvailBrkRgnTq_Nm/1 -> [VVMC_TotalAvailBrkRgnTq_Nm]
  Switch6/1 -> MSATorqueSourceDetermination/10(VTQD_SWCResUpSta_flg)  "VTQD_SWC2ResUpSta_flg"
  [VTQD_SWC2SetdownSta_flg] -> MSAActivationHandshake/8(VTQD_SWC2SetdownSta_flg)  "VTQD_SWC2SetdownSta_flg"
  [VTQD_SWC2ResUpSta_flg] -> MSAActivationHandshake/7(VTQD_SWC2ResUpSta_flg)  "VTQD_SWC2ResUpSta_flg"
  VTQD_SWC2ResUpSta_flg/1 -> [VTQD_SWC2ResUpSta_flg]
  VTQD_SWC2SetdownSta_flg/1 -> [VTQD_SWC2SetdownSta_flg]
  [VTQD_SpdCtrlMode_enum] -> MSAActivationHandshake/1(VTQD_SpdCtrlMode_enum)
  <VTQD_SpdCtrlMode_enum>/1 -> [VTQD_SpdCtrlMode_enum]
  Switch2/1 -> [VVMC_MSACtrlSta_enum]  "VVMC_MSACtrlSta_enum"
  Switch1/1 -> [VVMC_MSASpdWar_flg]  "VVMC_MSASpdWar_flg"
  Switch/1 -> [VVMC_MSAActive_flg]  "VVMC_MSAActive_flg"
  [VVMC_MSAActive_flg] -> MSADemandTorqueCalculation/3(VVMC_MSAActive_flg)
  MSADemandTorqueCalculation/1(VVMC_MSAWhlTqCal_Nm) -> [VVMC_MSAWhlTqCal_Nm]
  [VVMC_MSAWhlTqCal_Nm] -> MSATorqueSourceDetermination/1(VVMC_MSAWhlTqCal_Nm)
  MSATorqueSourceDetermination/1(VVMC_MSAWhlTqReq_Nm) -> [VVMC_MSAWhlTqReq_Nm]
  [VVMC_FeatArbitrFinal_enum] -> MSAActivationHandshake/2(VVMC_FeatArbitrFinal_enum)
  [VTQD_ExternalTqAllow_flg] -> MSAActivationHandshake/3(VTQD_ExternalTqAllow_flg)
  [VVMC_FeatSetSpdFinal_raw32] -> MSAActivationHandshake/5(VVMC_FeatSetSpdFinal_raw32)
  [VTQD_SWC2CANCELSta_flg] -> MSAActivationHandshake/6(VTQD_SWC2CANCELSta_flg)  "VTQD_SWC2CANCELSta_flg"
  [VVMC_FeatSetSpdForCalcu_kph] -> Switch3/3
  [VTQD_DriverWhlTqDem_Nm] -> MSATorqueSourceDetermination/2(VTQD_DriverWhlTqDem_Nm)
  VVMC_FeatArbitrFinal_enum/1 -> [VVMC_FeatArbitrFinal_enum]
  VTQD_ExternalTqAllow_flg/1 -> [VTQD_ExternalTqAllow_flg]
  VVMC_FeatSetSpdForCalcu_kph/1 -> Data Type Conversion/1
  VTQD_SWC2CANCELSta_flg/1 -> [VTQD_SWC2CANCELSta_flg]
  VTQD_DriverWhlTqDem_Nm/1 -> [VTQD_DriverWhlTqDem_Nm]
  [VVMC_MSACtrlSta_enum] -> VVMC_MSACtrlSta_enum/1
  [VVMC_MSASpdWar_flg] -> VVMC_MSASpdWar_flg/1
  [VVMC_MSAWhlTqReq_Nm] -> VVMC_MSAWhlTqReq_Nm/1
  Data Type Conversion/1 -> [VVMC_FeatSetSpdForCalcu_kph]  "VVMC_FeatSetSpdForCalcu_kph"
  [VVMC_MSAActive_flg] -> VVMC_MSAActive_flg/1
  VVMC_VehicleSpeed_kph/1 -> [VVMC_VehicleSpeed_kph]
  [VVMC_VehicleSpeed_kph] -> MSADemandTorqueCalculation/2(VVMC_VehicleSpeed_kph)
  [VVMC_MeterIndSpeed_raw32] -> MSAActivationHandshake/4(VVMC_MeterIndSpeed_raw32)
  VVMC_LongAcc_Gps/1 -> [VVMC_LongAcc_Gps]
  [VVMC_LongAcc_Gps] -> MSADemandTorqueCalculation/4(VVMC_LongAcc_Gps)
  VVMC_MeterIndSpeedForCalcu_kph/1 -> [VVMC_MeterIndSpeedForCalcu_kph]
  [VVMC_MeterIndSpeedForCalcu_kph] -> MSADemandTorqueCalculation/5(VVMC_MeterIndSpeedForCalcu_kph)
  VDHP_ActAPSPosn_pct/1 -> [VDHP_ActAPSPosn_pct]
  VTQD_LowIdleAccPedal_flg/1 -> [VTQD_LowIdleAccPedal_flg]
  [VTQD_LowIdleAccPedal_flg] -> MSATorqueSourceDetermination/3(VTQD_LowIdleAccPedal_flg)
  [VDHP_ActAPSPosn_pct] -> MSATorqueSourceDetermination/4(VDHP_ActAPSPosn_pct)
  [VVMC_VehicleSpeed_kph] -> MSATorqueSourceDetermination/5(VVMC_VehicleSpeed_kph)
  task_time_s/1 -> [task_time_s]
  [task_time_s] -> MSATorqueSourceDetermination/6(task_time_s)
  Switch4/1 -> MSATorqueSourceDetermination/7(VVMC_FeatSetSpdForCalcu_kph)
  VVMC_ActACCRequiredAccel_mps2/1 -> [VVMC_ActACCRequiredAccel_mps2]
  [VVMC_ActACCRequiredAccel_mps2] -> MSADemandTorqueCalculation/6(VVMC_ActACCRequiredAccel_mps2)
  VTQR_FrTMTqReq_Nm/1 -> [VTQR_FrTMTqReq_Nm]
  VTQR_RrTMTqReq_Nm/1 -> [VTQR_RrTMTqReq_Nm]
  [VTQR_FrTMTqReq_Nm] -> MSADemandTorqueCalculation/7(VTQR_FrTMTqReq_Nm)
  [VTQR_RrTMTqReq_Nm] -> MSADemandTorqueCalculation/8(VTQR_RrTMTqReq_Nm)
  [VVMC_MSAOvrdAllow_flg] -> MSADemandTorqueCalculation/9(VVMC_MSAPedalOvrd_flg)
  MSATorqueSourceDetermination/2(VVMC_MSAOvrdAllow_flg) -> [VVMC_MSAOvrdAllow_flg]
  [task_time_s] -> MSADemandTorqueCalculation/10(task_time_s)
  [VTQD_LowIdleAccPedal_flg] -> MSADemandTorqueCalculation/11(VTQD_LowIdleAccPedal_flg)
  [VVMC_MeterIndSpeedForCalcu_kph] -> MSATorqueSourceDetermination/8(VVMC_MeterIndSpeedForCalcu_kph)
  [VVMC_MSAOvrdAllow_flg] -> Unit Delay/1
  Unit Delay/1 -> MSAActivationHandshake/9(VVMC_MSAOvrdAllow_flg)
  [VVMC_MSAActive_flg] -> MSATorqueSourceDetermination/9(VVMC_MSAActive_flg)
  MSATorqueSourceDetermination/3(VVMC_MSAWhlTqActive_flg) -> [VVMC_MSAWhlTqActive_flg]
  [VVMC_MSAWhlTqActive_flg] -> VVMC_MSAWhlTqActive_flg/1
  VVMC_MeterIndSpeed_raw32/1 -> [VVMC_MeterIndSpeed_raw32]
  VINP_RDCActive_enum/1 -> [VINP_RDCActive_enum]
  [VINP_RDCActive_enum] -> MSADemandTorqueCalculation/13(VINP_RDCActive_enum)

== system vmc/VMC/VMC/PreConditionCheck ==
  VINP_DriverSeatBeltCmd_flg : Inport
  VBCM_DrDoorSW_flg : Inport  Port=2
  VTQD_GearActualPosn_enum : Inport  Port=3
  VINP_EPBSta_enum : Inport  Port=4
  VINP_ACCAvail_flg : Inport  Port=5
  VINP_AEBAvail_flg : Inport  Port=6
  VINP_ESCOFFStatus_enum : Inport  Port=7
  VINP_APSStaSystem_enum : Inport  Port=8
  VTQD_ExternalTqAllow_flg : Inport  Port=9
  VVMC_ACCCtrlAllow_flg : Inport  Port=10
  task_time_s : Inport  Port=11
  VDDM_VMCLongCtrlProhibited_flg : Inport  Port=12
  VDDM_LimpHomeAct_flg : Inport  Port=13
  VDDM_VCUMSAErr_flg : Inport  Port=14
  Cast To Single : DataTypeConversion  OutDataTypeStr=boolean
  Constant : Constant  Value=ENUM_DRDOORSW_CLOSE
  Constant1 : Constant  Value=ENUM_GEARACTUALPOSN_D
  Constant10 : Constant  Value=ENUM_APSSTASYSTEM_ACTIVE
  Constant11 : Constant  Value=ENUM_APSSTASYSTEM_REMOTEACTIVE
  Constant12 : Constant  Value=ENUM_EXTERNALTQALLOW_ALLOW
  Constant13 : Constant  Value=ENUM_ACCCTRLALLOW_ALLOW
  Constant14 : Constant  Value=ENUM_DRDOORSW_CLOSE
  Constant15 : Constant  Value=ENUM_GEARACTUALPOSN_D
  Constant16 : Constant  Value=KVMC_APSSWC_flg
  Constant17 : Constant  Value=ENUM_EPBSTA_RELEASED
  Constant18 : Constant  Value=ENUM_EXTERNALTQALLOW_ALLOW
  Constant{19,21,24,27,30} (5 alike) : Constant  Value=TRUE
  Constant{20,23,26,29} (4 alike) : Constant  Value=KVMC_PreCheckAllowTime_s
  Constant{22,25,28,31} (4 alike) : Constant  Value=FALSE
  Constant3 : Constant  Value=ENUM_EPBSTA_RELEASED
  Constant4 : Constant  Value=ENUM_ACCAVAIL_AVAILABLE
  Constant5 : Constant  Value=ENUM_AEBAVAIL_AVAILABLE
  Constant6 : Constant  Value=ENUM_ESCOFFSTATUS_NORMAL
  Constant7 : Constant  Value=ENUM_DRIVERSEATBELTCMD_LAMPOFF
  Constant8 : Constant  Value=ENUM_GEARACTUALPOSN_D
  Constant9 : Constant  Value=ENUM_GEARACTUALPOSN_N
  Logical Operator : Logic  AllPortsSameDT=off  OutDataTypeStr=boolean
  Logical Operator1 : Logic  Inputs=7  AllPortsSameDT=off  OutDataTypeStr=boolean
  Logical Operator2 : Logic  Inputs=3  AllPortsSameDT=off  OutDataTypeStr=boolean
  Logical Operator3 : Logic  Inputs=4  AllPortsSameDT=off  OutDataTypeStr=boolean
  Logical Operator4 : Logic  AllPortsSameDT=off  OutDataTypeStr=boolean
  Logical Operator5 : Logic  Inputs=7  AllPortsSameDT=off  OutDataTypeStr=boolean
  Logical Operator6 : Logic  Operator=OR  AllPortsSameDT=off  OutDataTypeStr=boolean
  NOT{,1..9} (10 alike) : Logic  Operator=NOT  AllPortsSameDT=off  OutDataTypeStr=boolean
  Relational Operator{,1,3..9,12..15,17..18} (15 alike) : RelationalOperator  Operator===  OutDataTypeStr=boolean  RndMeth=Simplest
  Relational Operator10 : RelationalOperator  Operator=~=  OutDataTypeStr=boolean  RndMeth=Simplest
  Relational Operator11 : RelationalOperator  Operator=~=  OutDataTypeStr=boolean  RndMeth=Simplest
  Relational Operator{16,19..21} (4 alike) : RelationalOperator  OutDataTypeStr=boolean  RndMeth=Simplest
  Timer{,1..3} (4 alike) : hcu_lib/Basic_Blocks/Timer
  u2 > 0 : Switch  Criteria=u2 > Threshold
  u2 > 0 (1){,1..3} (4 alike) : Switch  Criteria=u2 > Threshold
  VVMC_VMCACCCtrlAvail_flg : Outport
  VVMC_VMCAEBCtrlAvail_flg : Outport  Port=2
  VVMC_VMCCCCtrlAvail_flg : Outport  Port=3
  VVMC_VMCMSACtrlAvail_flg : Outport  Port=4
  wires:
  VDDM_VCUMSAErr_flg/1 -> [VDDM_VCUMSAErr_flg]
  VDDM_LimpHomeAct_flg/1 -> [VDDM_LimpHomeAct_flg]
  NOT8/1 -> Logical Operator5/7
  NOT9/1 -> Logical Operator5/6
  [VDDM_VCUMSAErr_flg] -> NOT9/1
  [VDDM_LimpHomeAct_flg] -> NOT8/1
  NOT7/1 -> Logical Operator1/5
  [VDDM_LimpHomeAct_flg] -> NOT7/1
  NOT6/1 -> Logical Operator5/5
  [VDDM_VMCLongCtrlProhibited_flg] -> NOT6/1
  NOT5/1 -> Logical Operator1/6
  [VDDM_VMCLongCtrlProhibited_flg] -> NOT5/1
  NOT4/1 -> Logical Operator3/4
  [VDDM_VMCLongCtrlProhibited_flg] -> NOT4/1
  VDDM_VMCLongCtrlProhibited_flg/1 -> [VDDM_VMCLongCtrlProhibited_flg]
  VBCM_DrDoorSW_flg/1 -> [VBCM_DrDoorSW_flg]
  VTQD_GearActualPosn_enum/1 -> [VTQD_GearActualPosn_enum]
  VINP_EPBSta_enum/1 -> [VINP_EPBSta_enum]
  VINP_ACCAvail_flg/1 -> [VINP_ACCAvail_flg]
  VINP_AEBAvail_flg/1 -> [VINP_AEBAvail_flg]
  VINP_ESCOFFStatus_enum/1 -> [VINP_ESCOFFStatus_enum]
  VINP_APSStaSystem_enum/1 -> [VINP_APSStaSystem_enum]
  Constant/1 -> Relational Operator/2
  [VBCM_DrDoorSW_flg] -> Relational Operator/1  "VBCM_DrDoorSW_flg"
  Constant1/1 -> Relational Operator1/2
  [VTQD_GearActualPosn_enum] -> Relational Operator1/1  "VTQD_GearActualPosn_enum"
  Constant3/1 -> Relational Operator3/2
  [VINP_EPBSta_enum] -> Relational Operator3/1  "VINP_EPBSta_enum"
  [VINP_ACCAvail_flg] -> Relational Operator4/1  "VINP_ACCAvail_flg"
  Constant4/1 -> Relational Operator4/2
  [VINP_AEBAvail_flg] -> Relational Operator5/1  "VINP_AEBAvail_flg"
  Constant5/1 -> Relational Operator5/2
  [VINP_ESCOFFStatus_enum] -> Relational Operator6/1  "VINP_ESCOFFStatus_enum"
  Constant6/1 -> Relational Operator6/2
  [VINP_APSStaSystem_enum] -> Relational Operator10/1
  Constant10/1 -> Relational Operator10/2
  [VINP_APSStaSystem_enum] -> Relational Operator11/1
  Constant11/1 -> Relational Operator11/2
  Relational Operator10/1 -> Logical Operator/1
  Relational Operator11/1 -> Logical Operator/2
  Relational Operator/1 -> Logical Operator1/1
  Relational Operator1/1 -> Logical Operator1/2
  Relational Operator3/1 -> Logical Operator1/3
  Relational Operator6/1 -> Logical Operator1/4
  Logical Operator/1 -> u2 > 0/1
  Relational Operator4/1 -> Logical Operator2/1
  Logical Operator1/1 -> Logical Operator4/1, Logical Operator2/3
  [VVMC_VMCAEBCtrlAvail_flg] -> VVMC_VMCAEBCtrlAvail_flg/1
  [VVMC_VMCACCCtrlAvail_flg] -> VVMC_VMCACCCtrlAvail_flg/1
  VTQD_ExternalTqAllow_flg/1 -> [VTQD_ExternalTqAllow_flg]
  Constant12/1 -> Relational Operator12/2
  [VTQD_ExternalTqAllow_flg] -> Relational Operator12/1
  Relational Operator12/1 -> Logical Operator4/2
  [VVMC_VMCCCCtrlAvail_flg] -> VVMC_VMCCCCtrlAvail_flg/1
  VVMC_ACCCtrlAllow_flg/1 -> [VVMC_ACCCtrlAllow_flg]
  Constant13/1 -> Relational Operator13/2
  [VVMC_ACCCtrlAllow_flg] -> Relational Operator13/1
  Relational Operator13/1 -> Logical Operator2/2
  [VINP_EPBSta_enum] -> Relational Operator17/1  "VINP_EPBSta_enum"
  Constant17/1 -> Relational Operator17/2
  [VTQD_GearActualPosn_enum] -> Relational Operator15/1  "VTQD_GearActualPosn_enum"
  Constant15/1 -> Relational Operator15/2
  [VBCM_DrDoorSW_flg] -> Relational Operator14/1  "VBCM_DrDoorSW_flg"
  Constant14/1 -> Relational Operator14/2
  [VTQD_ExternalTqAllow_flg] -> Relational Operator18/1
  Constant18/1 -> Relational Operator18/2
  Relational Operator14/1 -> Logical Operator5/1
  Relational Operator15/1 -> Logical Operator5/2
  Relational Operator17/1 -> Logical Operator5/3
  Relational Operator18/1 -> Logical Operator5/4
  [VVMC_VMCMSACtrlAvail_flg] -> VVMC_VMCMSACtrlAvail_flg/1
  VINP_DriverSeatBeltCmd_flg/1 -> [VINP_DriverSeatBeltCmd_flg]
  [VINP_DriverSeatBeltCmd_flg] -> Relational Operator7/1
  Constant7/1 -> Relational Operator7/2
  [VTQD_GearActualPosn_enum] -> Relational Operator8/1  "VTQD_GearActualPosn_enum"
  Constant8/1 -> Relational Operator8/2
  Constant9/1 -> Relational Operator9/2
  [VTQD_GearActualPosn_enum] -> Relational Operator9/1  "VTQD_GearActualPosn_enum"
  Relational Operator9/1 -> Logical Operator6/2
  Relational Operator8/1 -> Logical Operator6/1
  Logical Operator6/1 -> Logical Operator3/2
  Relational Operator7/1 -> Logical Operator3/1
  Relational Operator5/1 -> Logical Operator3/3
  Constant16/1 -> u2 > 0/2
  Constant19/1 -> u2 > 0/3
  u2 > 0/1 -> Cast To Single/1
  Cast To Single/1 -> Logical Operator1/7
  Constant22/1 -> u2 > 0 (1)/3
  [task_time_s] -> Timer/3
  Timer/1 -> Relational Operator16/1
  Relational Operator16/1 -> u2 > 0 (1)/2
  Constant20/1 -> Timer/4, Relational Operator16/2
  Constant21/1 -> u2 > 0 (1)/1
  NOT/1 -> Timer/2
  Logical Operator3/1 -> Timer/1, NOT/1
  u2 > 0 (1)/1 -> [VVMC_VMCAEBCtrlAvail_flg]  "VVMC_VMCAEBCtrlAvail_flg"
  task_time_s/1 -> [task_time_s]
  NOT1/1 -> Timer1/2
  Logical Operator2/1 -> Timer1/1, NOT1/1
  Constant24/1 -> u2 > 0 (1)1/1
  Constant23/1 -> Timer1/4, Relational Operator19/2
  Timer1/1 -> Relational Operator19/1
  Relational Operator19/1 -> u2 > 0 (1)1/2
  Constant25/1 -> u2 > 0 (1)1/3
  [task_time_s] -> Timer1/3
  u2 > 0 (1)1/1 -> [VVMC_VMCACCCtrlAvail_flg]  "VVMC_VMCACCCtrlAvail_flg"
  [task_time_s] -> Timer2/3
  Constant28/1 -> u2 > 0 (1)2/3
  Relational Operator20/1 -> u2 > 0 (1)2/2
  Timer2/1 -> Relational Operator20/1
  Constant26/1 -> Relational Operator20/2, Timer2/4
  Constant27/1 -> u2 > 0 (1)2/1
  Logical Operator4/1 -> NOT2/1, Timer2/1
  NOT2/1 -> Timer2/2
  u2 > 0 (1)2/1 -> [VVMC_VMCCCCtrlAvail_flg]  "VVMC_VMCCCCtrlAvail_flg"
  u2 > 0 (1)3/1 -> [VVMC_VMCMSACtrlAvail_flg]  "VVMC_VMCMSACtrlAvail_flg"
  NOT3/1 -> Timer3/2
  Logical Operator5/1 -> NOT3/1, Timer3/1
  Constant30/1 -> u2 > 0 (1)3/1
  Constant29/1 -> Timer3/4, Relational Operator21/2
  Timer3/1 -> Relational Operator21/1
  Relational Operator21/1 -> u2 > 0 (1)3/2
  Constant31/1 -> u2 > 0 (1)3/3
  [task_time_s] -> Timer3/3

== system vmc/VMC/VMC/RDC Determination ==
  task_time_s : Inport
  VVMC_ActMaxSlideRate_pct : Inport  Port=2
  VTQD_AfterAvailableTqDemFr_Nm : Inport  Port=3
  VTQD_AfterAvailableTqDemRr_Nm : Inport  Port=4
  VINP_ESCActive_flg : Inport  Port=5
  VINP_SASAngle_Deg : Inport  Port=6
  VINP_LatAccel_Gps : Inport  Port=7
  VVMC_VehicleSpeed_kph : Inport  Port=8
  VINP_YawRate_degps : Inport  Port=9
  VINP_RDCActive_enum : Inport  Port=10
  VINP_DIDGetDynoMode_flg : Inport  Port=11
  VINP_VehicleType_enum : Inport  Port=12
  VPMM_DrivetrainSelect_enum : Inport  Port=13
  RWD : Subsystem
  VVMC_RWDRDCActive_enum : Outport
  VVMC_RDCEnSlideRate_pct : Outport  Port=2
  VVMC_ActStESCYaw_degps : Outport  Port=3
  wires:
  [VPMM_DrivetrainSelect_enum] -> RWD/13(VPMM_DrivetrainSelect_enum)
  [VINP_VehicleType_enum] -> RWD/12(VINP_VehicleType_enum)
  VINP_VehicleType_enum/1 -> [VINP_VehicleType_enum]
  VPMM_DrivetrainSelect_enum/1 -> [VPMM_DrivetrainSelect_enum]
  VINP_LatAccel_Gps/1 -> [VINP_LatAccel_Gps]  "VINP_LatAccel_Gps"
  VINP_YawRate_degps/1 -> [VINP_YawRate_degps]  "VINP_YawRate_degps"
  [VINP_DIDGetDynoMode_flg] -> RWD/11(VINP_DIDGetDynoMode_flg)
  VINP_DIDGetDynoMode_flg/1 -> [VINP_DIDGetDynoMode_flg]
  [VVMC_ActStESCYaw_degps] -> VVMC_ActStESCYaw_degps/1
  [VVMC_RDCEnSlideRate_pct] -> VVMC_RDCEnSlideRate_pct/1
  RWD/3(VVMC_ActStESCYaw_Dps) -> [VVMC_ActStESCYaw_degps]
  RWD/2(VVMC_RDCEnSlideRate_pct) -> [VVMC_RDCEnSlideRate_pct]
  RWD/1(VVMC_RWDRDCActive_enum) -> [VVMC_RWDRDCActive_enum]
  VVMC_VehicleSpeed_kph/1 -> [VVMC_VehicleSpeed_kph]
  VINP_ESCActive_flg/1 -> [VINP_ESCActive_flg]
  VVMC_ActMaxSlideRate_pct/1 -> [VVMC_ActMaxSlideRate_pct]
  task_time_s/1 -> [task_time_s]
  VTQD_AfterAvailableTqDemRr_Nm/1 -> [VTQD_AfterAvailableTqDemRr_Nm]
  VINP_SASAngle_Deg/1 -> [VINP_SASAngle_Deg]
  VINP_RDCActive_enum/1 -> [VINP_RDCActive_enum]
  [VINP_ESCActive_flg] -> RWD/5(VINP_ESCActive_flg)
  [VTQD_AfterAvailableTqDemFr_Nm] -> RWD/3(VTQD_AfterAvailableTqDemFr_Nm)
  [task_time_s] -> RWD/1(task_time_s)
  [VINP_SASAngle_Deg] -> RWD/6(VINP_SASAngle_Deg)
  [VVMC_ActMaxSlideRate_pct] -> RWD/2(VVMC_ActMaxSlideRate_pct)
  [VINP_LatAccel_Gps] -> RWD/7(VINP_LatAccel_Gps)
  [VVMC_RWDRDCActive_enum] -> VVMC_RWDRDCActive_enum/1
  [VVMC_VehicleSpeed_kph] -> RWD/8(VVMC_VehicleSpeed_kph)
  [VINP_RDCActive_enum] -> RWD/10(VINP_RDCActive_enum)
  [VTQD_AfterAvailableTqDemRr_Nm] -> RWD/4(VTQD_AfterAvailableTqDemRr_Nm)
  VTQD_AfterAvailableTqDemFr_Nm/1 -> [VTQD_AfterAvailableTqDemFr_Nm]
  [VINP_YawRate_degps] -> RWD/9(VINP_YawRate_degps)
